simulink model "Hexa_CAD_quaternion_ANSFT"  (R2024b)
settings: Solver=ode4  StartTime=0.0  StopTime=60  FixedStep=0.01  RelTol=1e-3
model workspace (MAT data in the model file):
  hover_2m = [0 0 2 0 0 0 0 0 2 0 0 0 ... (36 elements, 6x6)]
  square = [0 0 2.5 0 0 0 0 0 2.5 0 0 0 ... (36 elements, 6x6)]
  tf : Simulink.Parameter (value not decoded)
  tray0 = [0 0 0 0 0 0 0.2 0.15 2 0 0 0 ... (36 elements, 6x6)]
  tray1 = [0 0 0 0 0 0 0 0 2 0 0 0 ... (36 elements, 6x6)]
  tray2 = [0 0 0 0 0 0 2 0 5 0 0 0 ... (36 elements, 6x6)]
  tray3 = [0 0 0 0 0 0 2 0 5 0 0 0 ... (36 elements, 6x6)]
  tray4 = [0 0 0 0 0 0 2 0 5 0.15 0 0 ... (36 elements, 6x6)]
  tray5 = [0 0 0 0 0 0 0 0 5 0.15 0 0 ... (36 elements, 6x6)]
  tray_yaw = [0 0 0 0 0 0 0 0 5 0 0 0 ... (36 elements, 6x6)]
undefined symbols (not defined in the file or in its folder): F, Light, MIL, smiData, X, Y, Z
libraries: sm_lib x167, nesl_utility x29, dspobslib x9, sharedtransform x4, simulink x4, aerolibutil x3, matrix_library x1, sharedutil x1, robotcorelib x1, aerolibwind2 x1
(part 6 of 6)

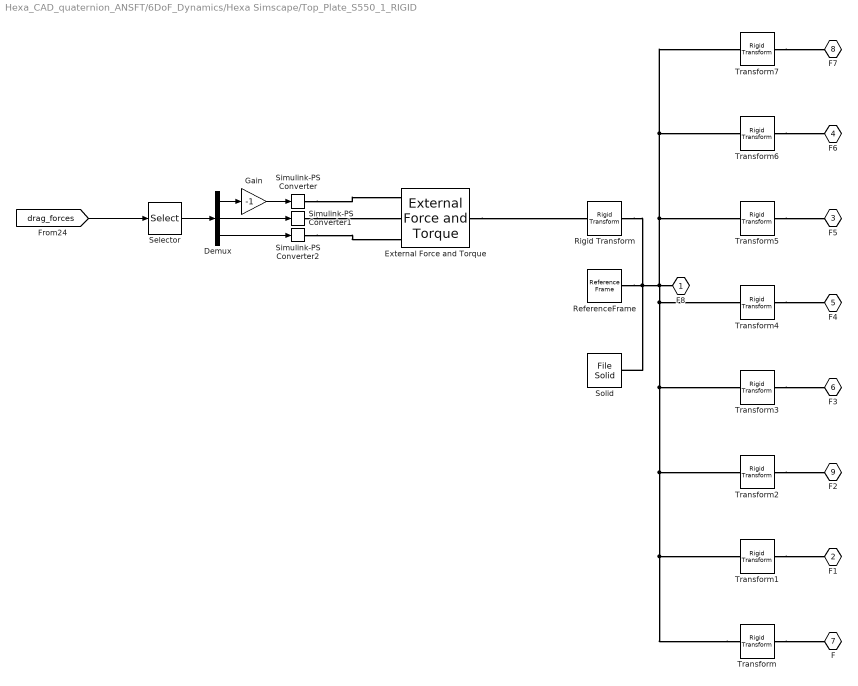
== system Hexa_CAD_quaternion_ANSFT/6DoF_Dynamics/Hexa Simscape/Top_Plate_S550_1_RIGID ==
  Demux : Demux  Outputs=3
  External Force and Torque : sm_lib/Forces and Torques/External Force and Torque  EnableForceX=on  EnableForceY=on  EnableForceZ=on  EnableForce=off  ForceResolutionFrame=AttachedFrame  EnableTorqueX=off  EnableTorqueY=off  EnableTorqueZ=off  EnableTorque=off  TorqueResolutionFrame=AttachedFrame
  Gain : Gain  Gain=-1
  ReferenceFrame : sm_lib/Frames and Transforms/Reference Frame
  Rigid Transform : sm_lib/Frames and Transforms/Rigid Transform  RotationMethod=None  FollAlignAxisA=+X  BaseAlignAxisA=+Y  FollAlignAxisB=+Y  BaseAlignAxisB=+Z  RotationStandardAxis=+Z  RotationAngle=0.0  RotationAngleUnits=deg  RotationArbitraryAxis=[0 0 1]  RotationSequenceAxes=FollowerAxes  RotationSequence=XYX  RotationSequenceAngles=[0 0 0]  RotationSequenceAnglesUnits=deg  RotationMatrix=[1 0 0; 0 1 0; 0 0 1]  Quaternion=[1 0 0 0]  TranslationMethod=None  TranslationCartesianOffset=[0 0 0]  TranslationCartesianOffsetUnits=m  TranslationStandardAxis=+Z  TranslationStandardOffset=0  TranslationStandardOffsetUnits=m  TranslationROffset=0  TranslationROffsetUnits=m  TranslationThetaOffset=0  TranslationThetaOffsetUnits=deg  TranslationZOffset=0  TranslationZOffsetUnits=m
  Selector : Selector  InputPortWidth=3  IndexOptions=Index vector (dialog)  Indices=[1 3 2]  OutputSizes=1
  Simulink-PS Converter : nesl_utility/Simulink-PS Converter  PhysicalDomain=network_engine_domain  SubClassName=ps_input  LeftPortType=input  RightPortType=output  PseudoPeriodic=off  Frequencies=[]  NoiseDistribution=none  NoiseParameters=[]  Unit=1  AffineConversion=off  FilteringAndDerivatives=provide  SimscapeFilterOrder=1  InputFilterTimeConstant=0.001  UdotUserProvided=0
  Simulink-PS Converter1 : nesl_utility/Simulink-PS Converter  PhysicalDomain=network_engine_domain  SubClassName=ps_input  LeftPortType=input  RightPortType=output  PseudoPeriodic=off  Frequencies=[]  NoiseDistribution=none  NoiseParameters=[]  Unit=1  AffineConversion=off  FilteringAndDerivatives=provide  SimscapeFilterOrder=1  InputFilterTimeConstant=0.001  UdotUserProvided=0
  Simulink-PS Converter2 : nesl_utility/Simulink-PS Converter  PhysicalDomain=network_engine_domain  SubClassName=ps_input  LeftPortType=input  RightPortType=output  PseudoPeriodic=off  Frequencies=[]  NoiseDistribution=none  NoiseParameters=[]  Unit=1  AffineConversion=off  FilteringAndDerivatives=provide  SimscapeFilterOrder=1  InputFilterTimeConstant=0.001  UdotUserProvided=0
  Solid : sm_lib/Body Elements/File Solid  ExtGeomFileName=Top_Plate_S550_Predeterminado_sldprt.STEP  UnitType=FromFile  ExtGeomFileUnits=m  StepReaderType=HEX  ExportConvexHullGeometry=off  InertiaType=Custom  BasedOnType=DensityFromFile  Density=1000  DensityUnits=kg/m^3  Mass=smiData.Solid(4).mass  MassUnits=kg  CenterOfMass=smiData.Solid(4).CoM  CenterOfMassUnits=mm  MomentsOfInertia=smiData.Solid(4).MoI  MomentsOfInertiaUnits=kg*mm^2  ProductsOfInertia=smiData.Solid(4).PoI  ProductsOfInertiaUnits=kg*mm^2  GraphicType=FromGeometry  MarkerShape=Sphere  MarkerSize=10  GraphicVisPropType=SimpleVisualProperties  GraphicDiffuseColor=[0.4 0.4 0.4]  GraphicOpacity=smiData.Solid(4).opacity  GraphicSpecularColor=[0.5 0.5 0.5 1.0]  GraphicAmbientColor=[0.15 0.15 0.15 1.0]  GraphicEmissiveColor=[0.0 0.0 0.0 1.0]  GraphicShininess=75  DoExposeReferenceFrame=on  SerializedFrames=<Frames/>
  Transform : sm_lib/Frames and Transforms/Rigid Transform  RotationMethod=ArbitraryAxis  FollAlignAxisA=+X  BaseAlignAxisA=+Y  FollAlignAxisB=+Y  BaseAlignAxisB=+Z  RotationStandardAxis=+Z  RotationAngle=smiData.RigidTransform(1).angle  RotationAngleUnits=rad  RotationArbitraryAxis=smiData.RigidTransform(1).axis  RotationSequenceAxes=FollowerAxes  RotationSequence=XYX  RotationSequenceAngles=[0 0 0]  RotationSequenceAnglesUnits=deg  RotationMatrix=[1 0 0; 0 1 0; 0 0 1]  Quaternion=[1 0 0 0]  TranslationMethod=Cartesian  TranslationCartesianOffset=smiData.RigidTransform(1).translation  TranslationCartesianOffsetUnits=mm  TranslationStandardAxis=+Z  TranslationStandardOffset=0  TranslationStandardOffsetUnits=m  TranslationROffset=0  TranslationROffsetUnits=m  TranslationThetaOffset=0  TranslationThetaOffsetUnits=deg  TranslationZOffset=0  TranslationZOffsetUnits=m
  Transform1 : sm_lib/Frames and Transforms/Rigid Transform  RotationMethod=ArbitraryAxis  FollAlignAxisA=+X  BaseAlignAxisA=+Y  FollAlignAxisB=+Y  BaseAlignAxisB=+Z  RotationStandardAxis=+Z  RotationAngle=smiData.RigidTransform(9).angle  RotationAngleUnits=rad  RotationArbitraryAxis=smiData.RigidTransform(9).axis  RotationSequenceAxes=FollowerAxes  RotationSequence=XYX  RotationSequenceAngles=[0 0 0]  RotationSequenceAnglesUnits=deg  RotationMatrix=[1 0 0; 0 1 0; 0 0 1]  Quaternion=[1 0 0 0]  TranslationMethod=Cartesian  TranslationCartesianOffset=smiData.RigidTransform(9).translation  TranslationCartesianOffsetUnits=mm  TranslationStandardAxis=+Z  TranslationStandardOffset=0  TranslationStandardOffsetUnits=m  TranslationROffset=0  TranslationROffsetUnits=m  TranslationThetaOffset=0  TranslationThetaOffsetUnits=deg  TranslationZOffset=0  TranslationZOffsetUnits=m
  Transform2 : sm_lib/Frames and Transforms/Rigid Transform  RotationMethod=ArbitraryAxis  FollAlignAxisA=+X  BaseAlignAxisA=+Y  FollAlignAxisB=+Y  BaseAlignAxisB=+Z  RotationStandardAxis=+Z  RotationAngle=smiData.RigidTransform(43).angle  RotationAngleUnits=rad  RotationArbitraryAxis=smiData.RigidTransform(43).axis  RotationSequenceAxes=FollowerAxes  RotationSequence=XYX  RotationSequenceAngles=[0 0 0]  RotationSequenceAnglesUnits=deg  RotationMatrix=[1 0 0; 0 1 0; 0 0 1]  Quaternion=[1 0 0 0]  TranslationMethod=Cartesian  TranslationCartesianOffset=smiData.RigidTransform(43).translation  TranslationCartesianOffsetUnits=mm  TranslationStandardAxis=+Z  TranslationStandardOffset=0  TranslationStandardOffsetUnits=m  TranslationROffset=0  TranslationROffsetUnits=m  TranslationThetaOffset=0  TranslationThetaOffsetUnits=deg  TranslationZOffset=0  TranslationZOffsetUnits=m
  Transform3 : sm_lib/Frames and Transforms/Rigid Transform  RotationMethod=ArbitraryAxis  FollAlignAxisA=+X  BaseAlignAxisA=+Y  FollAlignAxisB=+Y  BaseAlignAxisB=+Z  RotationStandardAxis=+Z  RotationAngle=smiData.RigidTransform(47).angle  RotationAngleUnits=rad  RotationArbitraryAxis=smiData.RigidTransform(47).axis  RotationSequenceAxes=FollowerAxes  RotationSequence=XYX  RotationSequenceAngles=[0 0 0]  RotationSequenceAnglesUnits=deg  RotationMatrix=[1 0 0; 0 1 0; 0 0 1]  Quaternion=[1 0 0 0]  TranslationMethod=Cartesian  TranslationCartesianOffset=smiData.RigidTransform(47).translation  TranslationCartesianOffsetUnits=mm  TranslationStandardAxis=+Z  TranslationStandardOffset=0  TranslationStandardOffsetUnits=m  TranslationROffset=0  TranslationROffsetUnits=m  TranslationThetaOffset=0  TranslationThetaOffsetUnits=deg  TranslationZOffset=0  TranslationZOffsetUnits=m
  Transform4 : sm_lib/Frames and Transforms/Rigid Transform  RotationMethod=ArbitraryAxis  FollAlignAxisA=+X  BaseAlignAxisA=+Y  FollAlignAxisB=+Y  BaseAlignAxisB=+Z  RotationStandardAxis=+Z  RotationAngle=smiData.RigidTransform(51).angle  RotationAngleUnits=rad  RotationArbitraryAxis=smiData.RigidTransform(51).axis  RotationSequenceAxes=FollowerAxes  RotationSequence=XYX  RotationSequenceAngles=[0 0 0]  RotationSequenceAnglesUnits=deg  RotationMatrix=[1 0 0; 0 1 0; 0 0 1]  Quaternion=[1 0 0 0]  TranslationMethod=Cartesian  TranslationCartesianOffset=smiData.RigidTransform(51).translation  TranslationCartesianOffsetUnits=mm  TranslationStandardAxis=+Z  TranslationStandardOffset=0  TranslationStandardOffsetUnits=m  TranslationROffset=0  TranslationROffsetUnits=m  TranslationThetaOffset=0  TranslationThetaOffsetUnits=deg  TranslationZOffset=0  TranslationZOffsetUnits=m
  Transform5 : sm_lib/Frames and Transforms/Rigid Transform  RotationMethod=ArbitraryAxis  FollAlignAxisA=+X  BaseAlignAxisA=+Y  FollAlignAxisB=+Y  BaseAlignAxisB=+Z  RotationStandardAxis=+Z  RotationAngle=smiData.RigidTransform(55).angle  RotationAngleUnits=rad  RotationArbitraryAxis=smiData.RigidTransform(55).axis  RotationSequenceAxes=FollowerAxes  RotationSequence=XYX  RotationSequenceAngles=[0 0 0]  RotationSequenceAnglesUnits=deg  RotationMatrix=[1 0 0; 0 1 0; 0 0 1]  Quaternion=[1 0 0 0]  TranslationMethod=Cartesian  TranslationCartesianOffset=smiData.RigidTransform(55).translation  TranslationCartesianOffsetUnits=mm  TranslationStandardAxis=+Z  TranslationStandardOffset=0  TranslationStandardOffsetUnits=m  TranslationROffset=0  TranslationROffsetUnits=m  TranslationThetaOffset=0  TranslationThetaOffsetUnits=deg  TranslationZOffset=0  TranslationZOffsetUnits=m
  Transform6 : sm_lib/Frames and Transforms/Rigid Transform  RotationMethod=ArbitraryAxis  FollAlignAxisA=+X  BaseAlignAxisA=+Y  FollAlignAxisB=+Y  BaseAlignAxisB=+Z  RotationStandardAxis=+Z  RotationAngle=smiData.RigidTransform(59).angle  RotationAngleUnits=rad  RotationArbitraryAxis=smiData.RigidTransform(59).axis  RotationSequenceAxes=FollowerAxes  RotationSequence=XYX  RotationSequenceAngles=[0 0 0]  RotationSequenceAnglesUnits=deg  RotationMatrix=[1 0 0; 0 1 0; 0 0 1]  Quaternion=[1 0 0 0]  TranslationMethod=Cartesian  TranslationCartesianOffset=smiData.RigidTransform(59).translation  TranslationCartesianOffsetUnits=mm  TranslationStandardAxis=+Z  TranslationStandardOffset=0  TranslationStandardOffsetUnits=m  TranslationROffset=0  TranslationROffsetUnits=m  TranslationThetaOffset=0  TranslationThetaOffsetUnits=deg  TranslationZOffset=0  TranslationZOffsetUnits=m
  Transform7 : sm_lib/Frames and Transforms/Rigid Transform  RotationMethod=ArbitraryAxis  FollAlignAxisA=+X  BaseAlignAxisA=+Y  FollAlignAxisB=+Y  BaseAlignAxisB=+Z  RotationStandardAxis=+Z  RotationAngle=smiData.RigidTransform(63).angle  RotationAngleUnits=rad  RotationArbitraryAxis=smiData.RigidTransform(63).axis  RotationSequenceAxes=FollowerAxes  RotationSequence=XYX  RotationSequenceAngles=[0 0 0]  RotationSequenceAnglesUnits=deg  RotationMatrix=[1 0 0; 0 1 0; 0 0 1]  Quaternion=[1 0 0 0]  TranslationMethod=Cartesian  TranslationCartesianOffset=smiData.RigidTransform(63).translation  TranslationCartesianOffsetUnits=mm  TranslationStandardAxis=+Z  TranslationStandardOffset=0  TranslationStandardOffsetUnits=m  TranslationROffset=0  TranslationROffsetUnits=m  TranslationThetaOffset=0  TranslationThetaOffsetUnits=deg  TranslationZOffset=0  TranslationZOffsetUnits=m
  F8 : PMIOPort  Side=Left
  F1 : PMIOPort  Port=2  Side=Left
  F5 : PMIOPort  Port=3  Side=Left
  F6 : PMIOPort  Port=4  Side=Left
  F4 : PMIOPort  Port=5  Side=Right
  F3 : PMIOPort  Port=6  Side=Right
  F : PMIOPort  Port=7  Side=Right
  F7 : PMIOPort  Port=8  Side=Right
  F2 : PMIOPort  Port=9  Side=Right
  wires:
  [drag_forces] -> Selector/1
  Selector/1 -> Demux/1
  Demux/1 -> Gain/1
  Demux/2 -> Simulink-PS Converter1/1
  Demux/3 -> Simulink-PS Converter2/1
  Gain/1 -> Simulink-PS Converter/1
  connections:
  Transform/LConn1 -- Transform1/LConn1 -- Transform6/LConn1 -- Transform7/LConn1 -- Transform5/LConn1 -- Rigid Transform/LConn1 -- ReferenceFrame/RConn1 -- Solid/RConn1 -- F8/RConn1 -- Transform4/LConn1 -- Transform3/LConn1 -- Transform2/LConn1
  Transform/RConn1 -- F/RConn1
  Transform1/RConn1 -- F1/RConn1
  Transform2/RConn1 -- F2/RConn1
  Transform3/RConn1 -- F3/RConn1
  Transform4/RConn1 -- F4/RConn1
  Transform5/RConn1 -- F5/RConn1
  Transform6/RConn1 -- F6/RConn1
  Transform7/RConn1 -- F7/RConn1
  External Force and Torque/RConn1 -- Rigid Transform/RConn1
  Simulink-PS Converter/RConn1 -- External Force and Torque/LConn1
  Simulink-PS Converter1/RConn1 -- External Force and Torque/LConn2
  Simulink-PS Converter2/RConn1 -- External Force and Torque/LConn3

== system Hexa_CAD_quaternion_ANSFT/6DoF_Dynamics/Hexa Simscape/Turnigy_5000mAh_3S_1_RIGID ==
  ReferenceFrame : sm_lib/Frames and Transforms/Reference Frame
  Solid : sm_lib/Body Elements/File Solid  ExtGeomFileName=Turnigy 5000mAh 3S_Predeterminado_sldprt.STEP  UnitType=FromFile  ExtGeomFileUnits=m  StepReaderType=HEX  ExportConvexHullGeometry=off  InertiaType=Custom  BasedOnType=DensityFromFile  Density=1000  DensityUnits=kg/m^3  Mass=smiData.Solid(10).mass  MassUnits=kg  CenterOfMass=smiData.Solid(10).CoM  CenterOfMassUnits=mm  MomentsOfInertia=smiData.Solid(10).MoI  MomentsOfInertiaUnits=kg*mm^2  ProductsOfInertia=smiData.Solid(10).PoI  ProductsOfInertiaUnits=kg*mm^2  GraphicType=FromGeometry  MarkerShape=Sphere  MarkerSize=10  GraphicVisPropType=SimpleVisualProperties  GraphicDiffuseColor=smiData.Solid(10).color  GraphicOpacity=smiData.Solid(10).opacity  GraphicSpecularColor=[0.5 0.5 0.5 1.0]  GraphicAmbientColor=[0.15 0.15 0.15 1.0]  GraphicEmissiveColor=[0.0 0.0 0.0 1.0]  GraphicShininess=75  DoExposeReferenceFrame=on  SerializedFrames=<Frames/>
  Transform : sm_lib/Frames and Transforms/Rigid Transform  RotationMethod=ArbitraryAxis  FollAlignAxisA=+X  BaseAlignAxisA=+Y  FollAlignAxisB=+Y  BaseAlignAxisB=+Z  RotationStandardAxis=+Z  RotationAngle=smiData.RigidTransform(14).angle  RotationAngleUnits=rad  RotationArbitraryAxis=smiData.RigidTransform(14).axis  RotationSequenceAxes=FollowerAxes  RotationSequence=XYX  RotationSequenceAngles=[0 0 0]  RotationSequenceAnglesUnits=deg  RotationMatrix=[1 0 0; 0 1 0; 0 0 1]  Quaternion=[1 0 0 0]  TranslationMethod=Cartesian  TranslationCartesianOffset=smiData.RigidTransform(14).translation  TranslationCartesianOffsetUnits=mm  TranslationStandardAxis=+Z  TranslationStandardOffset=0  TranslationStandardOffsetUnits=m  TranslationROffset=0  TranslationROffsetUnits=m  TranslationThetaOffset=0  TranslationThetaOffsetUnits=deg  TranslationZOffset=0  TranslationZOffsetUnits=m
  F : PMIOPort  Side=Left
  connections:
  ReferenceFrame/RConn1 -- Solid/RConn1 -- Transform/LConn1
  Transform/RConn1 -- F/RConn1

== matlab function Hexa_CAD_quaternion_ANSFT/Controller/Kronecker product6/Kronecker_product ==
  data: q input; r output; p input
function r = fcn(q, p)

%{
    Function to describe in matrix math the Kronecker product between
    two quaternions
    
    r = p kronecker q
    %}

    len = length(p);

    if len == 3
        p1 = [0; p];
        q0 = q(1);
        q1 = q(2);
        q2 = q(3);
        q3 = q(4);
        
        % skew symmetric matrix
        q_matrix = [q0, -q1, -q2, -q3;
                  q1, q0, -q3, q2;
                  q2, q3, q0, -q1;
                  q3, -q2, q1, q0];
        
        r = q_matrix * p1;

    elseif len == 4
        q0 = q(1);
        q1 = q(2);
        q2 = q(3);
        q3 = q(4);
        
        % skew symmetric matrix
        q_matrix = [q0, -q1, -q2, -q3;
                  q1, q0, -q3, q2;
                  q2, q3, q0, -q1;
                  q3, -q2, q1, q0];
        
        r = q_matrix * p;

    else
        error('Quaternions dimensions do not match')
    end

== matlab function Hexa_CAD_quaternion_ANSFT/Controller/Kronecker product7/Kronecker_product ==
  data: q input; r output; p input
function r = fcn(q, p)

%{
    Function to describe in matrix math the Kronecker product between
    two quaternions
    
    r = p kronecker q
    %}

    len = length(p);

    if len == 3
        p1 = [0; p];
        q0 = q(1);
        q1 = q(2);
        q2 = q(3);
        q3 = q(4);
        
        % skew symmetric matrix
        q_matrix = [q0, -q1, -q2, -q3;
                  q1, q0, -q3, q2;
                  q2, q3, q0, -q1;
                  q3, -q2, q1, q0];
        
        r = q_matrix * p1;

    elseif len == 4
        q0 = q(1);
        q1 = q(2);
        q2 = q(3);
        q3 = q(4);
        
        % skew symmetric matrix
        q_matrix = [q0, -q1, -q2, -q3;
                  q1, q0, -q3, q2;
                  q2, q3, q0, -q1;
                  q3, -q2, q1, q0];
        
        r = q_matrix * p;

    else
        error('Quaternions dimensions do not match')
    end

== matlab function Hexa_CAD_quaternion_ANSFT/Controller/ANSFT Constants ==
  data: xi1 output; xi2 output; lambda1 output; lambda2 output; alpha output; beta output; epsilon output
function [xi1, xi2, lambda1, lambda2, alpha, beta, epsilon] = fcn

% %% Constantes de la Superficie deslizante
% xi1 = [2.5; 2.5; 1.5; 1; 1; 1];
% xi2 = [1.25; 1.25; 2; 0.5; 0.5; 0.5];
% lambda1 = [1.5; 1.5; 1.75; 2; 2; 2];
% lambda2 = [1.2; 1.2; 1.25; 1.2; 1.2; 1.2];
% %% Constantes del control auxiliar
% alpha = [1.75; 1.75; 0.625; 2.5; 2.5; 1.5];
% beta = [2.5; 2.5; 0.1; 0.05; 0.05; 5];
% epsilon = [0.4; 0.4; 0.4; 0.4; 0.4; 0.4];

%% Constantes de la Superficie deslizante
xi1 = [2.5; 2.5; 1.5; 1; 1; 1];
xi2 = [1.25; 1.25; 2; 0.5; 0.5; 0.5];
lambda1 = [1.5; 1.5; 1.75; 2; 2; 2];
lambda2 = [1.2; 1.2; 1.25; 1.2; 1.2; 1.2];
%% Constantes del control auxiliar
alpha = [1.75; 1.75; 0.625; 2.5; 2.5; 1.25];
beta = [2.5; 2.5; 0.1; 0.05; 0.05; 0.25];
epsilon = [0.4; 0.4; 0.4; 0.4; 0.4; 0.4];

== matlab function Hexa_CAD_quaternion_ANSFT/Controller/Constants Functions ==
  data: J output; g output; m output
function [J, g, m]  = fcn

%% system constants
% m = 1.52; %5 mass 2.2 kg
Jxx = 0.03;       % Inercia x.
Jyy = 0.03;       % Inercia y.
Jzz = 0.05;       % Inercia z.

J = diag([Jxx, Jyy, Jzz]);

g = [0; 0; -9.81];

m = 1.57;

== matlab function Hexa_CAD_quaternion_ANSFT/6DoF_Dynamics/calculatePWM ==
  data: omega2 input; pwm output
function pwm = fcn(omega2)

pwm = -1.935e-09 .* omega2 .* omega2 + 0.001723 .* omega2 + 1114.0412;

== matlab function Hexa_CAD_quaternion_ANSFT/Trajectory/Kronecker product5/Kronecker_product ==
  data: q input; r output size=[4 1]; p input
function r = fcn(q, p)

%{
    Function to describe in matrix math the Kronecker product between
    two quaternions
    
    r = p kronecker q
    %}

    len = length(p);

    if len == 3 && length(q) == 4
        p1 = [0; p];
        q0 = q(1);
        q1 = q(2);
        q2 = q(3);
        q3 = q(4);
        
        % skew symmetric matrix
        q_matrix = [q0, -q1, -q2, -q3;
                  q1, q0, -q3, q2;
                  q2, q3, q0, -q1;
                  q3, -q2, q1, q0];
        
        r = q_matrix * p1;

    elseif len == 4
        q0 = q(1);
        q1 = q(2);
        q2 = q(3);
        q3 = q(4);
        
        % skew symmetric matrix
        q_matrix = [q0, -q1, -q2, -q3;
                  q1, q0, -q3, q2;
                  q2, q3, q0, -q1;
                  q3, -q2, q1, q0];
        
        r = q_matrix * p;

    else
        error('Quaternions dimensions do not match')
    end

== matlab function Hexa_CAD_quaternion_ANSFT/Trajectory/Helicoidal Trajectory ==
  data: time input; pose_d output; pose_d_dot output; pose_d_ddot output
function [pose_d, pose_d_dot, pose_d_ddot]= fcn(time)

% pos_z = time / 12;
f = 0.15;
arg = f * (time - 5);
r = 2;

% hover for 5 s | include inclination in roll
% 5 metros al menos

if (time < 5)
    pos_x = 0;
    pos_y = 0;
    % roll = 0;
    pos_z = 0.4 * time;
else
    pos_x = -r + r * cos (arg);
    pos_y = r * sin (arg);
    pos_z = 2;
end

% roll = 0;
% yaw = time * 0;

pose_d = [pos_x;
          pos_y;
          pos_z];
          % roll;
          % 0;
          % yaw];

% pos_z_dot = 1 / 12;

% hover for 5 s
if (time < 5)
    pos_x_dot = 0;
    pos_y_dot = 0;
    pos_z_dot = 0.4;
else
    pos_x_dot = - f * r * sin(arg);
    pos_y_dot = f * r * cos(arg);
    pos_z_dot= 0;
end

% yaw_dot = 0;

pose_d_dot = [pos_x_dot;
              pos_y_dot;
              pos_z_dot];
              % 0;
              % 0;
              % yaw_dot];

pos_z_ddot = 0;
% hover for 5 s
if (time < 5)
    pos_x_ddot = 0;
    pos_y_ddot = 0;
else
    pos_x_ddot = - f * f * r * cos(arg);
    pos_y_ddot = - f * f * r * sin(arg);
end

% yaw_ddot = 0;

pose_d_ddot = [pos_x_ddot;
               pos_y_ddot;
               pos_z_ddot];
               % 0;
               % 0;
               % yaw_ddot];

== matlab function Hexa_CAD_quaternion_ANSFT/Trajectory/Lemniscate Trajectory ==
  data: time input; pose_d output; pose_d_dot output; pose_d_ddot output
function [pose_d, pose_d_dot, pose_d_ddot] = fcn(time)

%% Positions

arg = time / 4;

pos_x = cos(arg) ./ (1 + sin(arg) .* sin(arg));
pos_y = cos(arg) .* sin(arg) ./ (1 + sin(arg) .* sin(arg));
pos_z = sin(arg);

% yaw = time * 0;

pose_d = [pos_x;
          pos_y;
          pos_z];
          % 0;
          % 0;
          % yaw];

%% Velocities

pos_z_dot = 0.25 * cos(arg);
pos_x_dot = - sin(arg)/(4*(sin(arg)^2 + 1)) - (cos(arg)^2*sin(arg))/(2*(sin(arg)^2 + 1)^2);
pos_y_dot = cos(arg)^2/(4*(sin(arg)^2 + 1)) - sin(arg)^2/(4*(sin(arg)^2 + 1)) - (cos(arg)^2*sin(arg)^2)/(2*(sin(arg)^2 + 1)^2);
% yaw_dot = 0;

pose_d_dot = [pos_x_dot;
              pos_y_dot;
              pos_z_dot];
              % 0;
              % 0;
              % yaw_dot];

%% Accelerations

pos_z_ddot = -0.25 * 0.25 * sin(arg);
pos_x_ddot = 0;
pos_y_ddot = 0;
% yaw_ddot = 0;

pose_d_ddot = [pos_x_ddot;
               pos_y_ddot;
               pos_z_ddot];
               % 0;
               % 0;
               % yaw_ddot];

== matlab function Hexa_CAD_quaternion_ANSFT/Trajectory/Kronecker product3/Kronecker_product ==
  data: q input; r output size=[4 1]; p input
function r = fcn(q, p)

%{
    Function to describe in matrix math the Kronecker product between
    two quaternions
    
    r = p kronecker q
    %}

    len = length(p);

    if len == 3 && length(q) == 4
        p1 = [0; p];
        q0 = q(1);
        q1 = q(2);
        q2 = q(3);
        q3 = q(4);
        
        % skew symmetric matrix
        q_matrix = [q0, -q1, -q2, -q3;
                  q1, q0, -q3, q2;
                  q2, q3, q0, -q1;
                  q3, -q2, q1, q0];
        
        r = q_matrix * p1;

    elseif len == 4
        q0 = q(1);
        q1 = q(2);
        q2 = q(3);
        q3 = q(4);
        
        % skew symmetric matrix
        q_matrix = [q0, -q1, -q2, -q3;
                  q1, q0, -q3, q2;
                  q2, q3, q0, -q1;
                  q3, -q2, q1, q0];
        
        r = q_matrix * p;

    else
        error('Quaternions dimensions do not match')
    end

== matlab function Hexa_CAD_quaternion_ANSFT/Controller/quaterniontoPRV/MATLAB Function ==
  data: q input; lnq output size=[3 1]
function lnq = fcn(q)

if length(q) == 4
    q0 = q(1);
    q_vec = [q(2); q(3); q(4)];

    if norm(q_vec) == 0
        lnq = [0; 0; 0];
    else
        % q0 = real(q0);
        lnq = (q_vec / (norm(q_vec)) ) * acos(q0);
    end
else
    error('Input must be a vector 4 by 1 (Quaternion)')
end

== matlab function Hexa_CAD_quaternion_ANSFT/Trajectory/calculateAttitudeTrajectory ==
  data: qx output; qy output; t input; qz output; w_d output; w_d_dot output
function [qx, qy, qz, w_d, w_d_dot] = fcn(t)

roll = 0.0;
pitch = 0.0;
% yaw = 90 * pi / 180;
f = 0.15;
p = 40 * pi / 3 + 5;

if t < 5
    % roll = 0;
    % roll_d = 0;
    % pitch = 0;
    yaw = 0;
    w_d = [0; 0; 0];
else
    % roll = 5 * pi / 180 * sin(t - 5);
    % roll_d = 5 * pi / 180 * cos(t - 5);
    yaw = 2 * pi * (t - 5)/ (p - 5);
    w_d = [0; 0; 2 * pi / (p - 5)];
    % w_d = [0; 0; 0];
    % w_d = [roll_d; 0; 0];
end

qx = [cos(roll/2);
      sin(roll/2);
      0;
      0];

qy = [cos(pitch/2);
      0;
      sin(pitch/2);
      0];

qz = [cos(yaw/2);
      0;
      0;
      sin(yaw/2)];

% w_d = [0; 0; 0];
w_d_dot = [0; 0; 0];

== matlab function Hexa_CAD_quaternion_ANSFT/Controller/Kronecker product4/Kronecker_product ==
  data: q input; r output size=[4 1]; p input
function r = fcn(q, p)

%{
    Function to describe in matrix math the Kronecker product between
    two quaternions
    
    r = p kronecker q
    %}

    len = length(p);

    if len == 3 && length(q) == 4
        p1 = [0; p];
        q0 = q(1);
        q1 = q(2);
        q2 = q(3);
        q3 = q(4);
        
        % skew symmetric matrix
        q_matrix = [q0, -q1, -q2, -q3;
                  q1, q0, -q3, q2;
                  q2, q3, q0, -q1;
                  q3, -q2, q1, q0];
        
        r = q_matrix * p1;

    elseif len == 4
        q0 = q(1);
        q1 = q(2);
        q2 = q(3);
        q3 = q(4);
        
        % skew symmetric matrix
        q_matrix = [q0, -q1, -q2, -q3;
                  q1, q0, -q3, q2;
                  q2, q3, q0, -q1;
                  q3, -q2, q1, q0];
        
        r = q_matrix * p;

    else
        error('Quaternions dimensions do not match')
    end
